simulink model "SVPWM_FOC"  (R2024a)
settings: Solver=ode23tb  StartTime=0.0  StopTime=1  MaxStep=0.00001  RelTol=1e-3
libraries: spsVoltageMeasurementLib x6, spsMosfetLib x6, slpidlib x3, spsDCVoltageSourceLib x2, spsPermanentMagnetSynchronousMachineLib x1, simulink x1, autolibpmsmexterior x1, spsUniversalBridgeLib x1, sps_lib x1
settings Model: Creator=hzn  LastModifiedBy=hzn

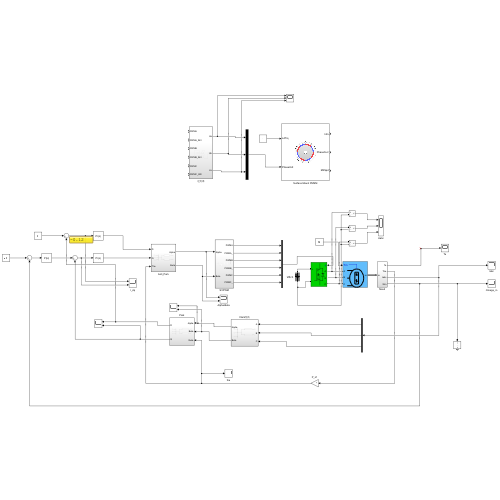
[thumbnail: Simulink's stored preview of the top-level diagram]
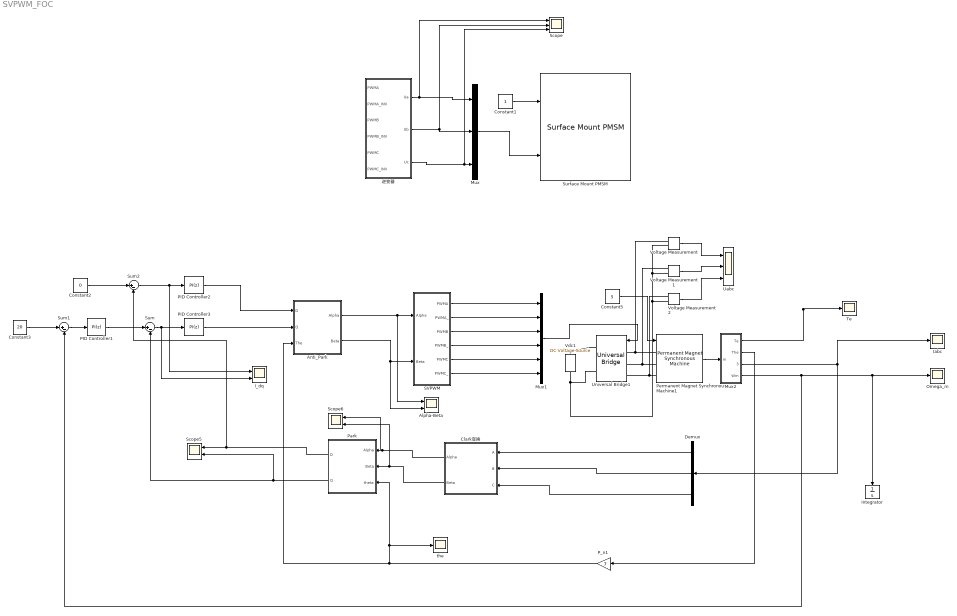
== system SVPWM_FOC ==
  Alpha-Beta : Scope  NumInputPorts=2
  Anti_Park : Subsystem
  Clark变换 : Subsystem
  Constant1 : Constant
  Constant2 : Constant  Value=0
  Constant3 : Constant  Value=20
  Constant5 : Constant  Value=5
  Demux : Demux  Outputs=3
  I_dq : Scope  NumInputPorts=2
  Iabc : Scope
  Integrator : Integrator
  Mux : Mux  Inputs=3
  Mux1 : Mux  Inputs=6
  Mux2 : Subsystem
  Omega_m : Scope
  PID Controller1 : slpidlib/PID Controller  Controller=PI  Form=Parallel  TimeDomain=Discrete-time  UseExternalTs=off  SampleTime=-1  IntegratorMethod=Forward Euler  FilterMethod=Forward Euler  ControllerParametersSource=internal  P=0.7  I=35  UseKiTs=off  D=0  UseExternalDerivativeSource=off  N=100  UseFilter=on  TunerSelectOption=Transfer Function Based (PID Tuner App)  InitialConditionSource=internal  InitialConditionForIntegrator=0  InitialConditionForFilter=0  DifferentiatorICPrevScaledInput=0  ExternalReset=none  TrackingMode=off  Kt=1  LimitOutput=off  SatLimitsSource=internal  UpperSaturationLimit=inf  LowerSaturationLimit=-inf  LinearizeAsGain=on  AntiWindupMode=none  Kb=1  LimitIntegrator=off  UpperIntegratorSaturationLimit=inf  LowerIntegratorSaturationLimit=-inf  POutMin=[]  POutMax=[]  IOutMin=[]  IOutMax=[]  DOutMin=[]  DOutMax=[]  NOutMin=[]  NOutMax=[]  SumOutMin=[]  SumOutMax=[]  SaturationOutMin=[]  SaturationOutMax=[]  PParamMin=[]  PParamMax=[]  IParamMin=[]  IParamMax=[]  DParamMin=[]  DParamMax=[]  NParamMin=[]  NParamMax=[]  KbParamMin=[]  KbParamMax=[]  KtParamMin=[]  KtParamMax=[]  KbOutMin=[]  KbOutMax=[]  KtOutMin=[]  KtOutMax=[]  IntegratorOutMin=[]  IntegratorOutMax=[]  FilterOutMin=[]  FilterOutMax=[]  SumI1OutMin=[]  SumI1OutMax=[]  SumI2OutMin=[]  SumI2OutMax=[]  SumI3OutMin=[]  SumI3OutMax=[]  SumI4OutMin=[]  SumI4OutMax=[]  SumDOutMin=[]  SumDOutMax=[]  DifferentiatorOutMin=[]  DifferentiatorOutMax=[]  FilterDiffOutCoefMin=[]  FilterDiffOutCoefMax=[]  ReciprocalOutMin=[]  ReciprocalOutMax=[]  SumDenOutMin=[]  SumDenOutMax=[]  SumNumOutMin=[]  SumNumOutMax=[]  DivideOutMin=[]  DivideOutMax=[]  UdiffTsProdOutMin=[]  UdiffTsProdOutMax=[]  NTsProdOutMin=[]  NTsProdOutMax=[]  UintegralTsProdOutMin=[]  UintegralTsProdOutMax=[]  UngainTsProdOutMin=[]  UngainTsProdOutMax=[]  ClampingZeroOutDataTypeStr=Inherit: Inherit via back propagation  ClampingZeroOutMin=[]  ClampingZeroOutMax=[]  FilterDenConstantOutDataTypeStr=Inherit: Inherit via back propagation  FilterDenConstantOutMin=[]  FilterDenConstantOutMax=[]  PCopyOutDataTypeStr=Inherit: Inherit via back propagation  PCopyOutMin=[]  PCopyOutMax=[]  NCopyOutDataTypeStr=Inherit: Inherit via back propagation  NCopyOutMin=[]  NCopyOutMax=[]  IntegratorContinuousStateAttributes=''  IntegratorStateMustResolveToSignalObject=off  IntegratorRTWStateStorageClass=Auto  FilterContinuousStateAttributes=''  FilterStateMustResolveToSignalObject=off  FilterRTWStateStorageClass=Auto  ParallelPVariant=InternalParameters  IdealPVariant=Disabled  IVariant=InternalParameters  DVariant=Disabled  IntegratorVariant=Discrete  SatVariant=Disabled  AWVariant=Passthrough  PCopyVariant=Disabled  TRVariant=Disabled  FdbkBlocksVariant=Forward  IdealPFdbkVariant=Disabled  SatFdbkVariant=Disabled  DerivativeFilterVariant=Disabled  NVariant=Disabled  NCopyVariant=Disabled_SignalSpec  FilterICVariant=Disabled  IntegratorICVariant=InternalICs  ExternalResetVariant=Disabled  TRSumVariant=Passthrough  SumFdbkVariant=Disabled  SumVariant=Sum_PI  TsampFilterVariant=InternalTs  TsampNgainVariant=Passthrough  TsampIntegralVariant=Disabled_SignalSpec  ExternalSaturationOutDataTypeStr=Inherit: Same as second input  DerivativeSourceVariant=Disabled
  PID Controller2 : slpidlib/PID Controller  Controller=PI  Form=Parallel  TimeDomain=Discrete-time  UseExternalTs=off  SampleTime=-1  IntegratorMethod=Forward Euler  FilterMethod=Forward Euler  ControllerParametersSource=internal  P=5  I=80  UseKiTs=off  D=0  UseExternalDerivativeSource=off  N=100  UseFilter=on  TunerSelectOption=Transfer Function Based (PID Tuner App)  InitialConditionSource=internal  InitialConditionForIntegrator=0  InitialConditionForFilter=0  DifferentiatorICPrevScaledInput=0  ExternalReset=none  TrackingMode=off  Kt=1  LimitOutput=off  SatLimitsSource=internal  UpperSaturationLimit=inf  LowerSaturationLimit=-inf  LinearizeAsGain=on  AntiWindupMode=none  Kb=1  LimitIntegrator=off  UpperIntegratorSaturationLimit=inf  LowerIntegratorSaturationLimit=-inf  POutMin=[]  POutMax=[]  IOutMin=[]  IOutMax=[]  DOutMin=[]  DOutMax=[]  NOutMin=[]  NOutMax=[]  SumOutMin=[]  SumOutMax=[]  SaturationOutMin=[]  SaturationOutMax=[]  PParamMin=[]  PParamMax=[]  IParamMin=[]  IParamMax=[]  DParamMin=[]  DParamMax=[]  NParamMin=[]  NParamMax=[]  KbParamMin=[]  KbParamMax=[]  KtParamMin=[]  KtParamMax=[]  KbOutMin=[]  KbOutMax=[]  KtOutMin=[]  KtOutMax=[]  IntegratorOutMin=[]  IntegratorOutMax=[]  FilterOutMin=[]  FilterOutMax=[]  SumI1OutMin=[]  SumI1OutMax=[]  SumI2OutMin=[]  SumI2OutMax=[]  SumI3OutMin=[]  SumI3OutMax=[]  SumI4OutMin=[]  SumI4OutMax=[]  SumDOutMin=[]  SumDOutMax=[]  DifferentiatorOutMin=[]  DifferentiatorOutMax=[]  FilterDiffOutCoefMin=[]  FilterDiffOutCoefMax=[]  ReciprocalOutMin=[]  ReciprocalOutMax=[]  SumDenOutMin=[]  SumDenOutMax=[]  SumNumOutMin=[]  SumNumOutMax=[]  DivideOutMin=[]  DivideOutMax=[]  UdiffTsProdOutMin=[]  UdiffTsProdOutMax=[]  NTsProdOutMin=[]  NTsProdOutMax=[]  UintegralTsProdOutMin=[]  UintegralTsProdOutMax=[]  UngainTsProdOutMin=[]  UngainTsProdOutMax=[]  ClampingZeroOutDataTypeStr=Inherit: Inherit via back propagation  ClampingZeroOutMin=[]  ClampingZeroOutMax=[]  FilterDenConstantOutDataTypeStr=Inherit: Inherit via back propagation  FilterDenConstantOutMin=[]  FilterDenConstantOutMax=[]  PCopyOutDataTypeStr=Inherit: Inherit via back propagation  PCopyOutMin=[]  PCopyOutMax=[]  NCopyOutDataTypeStr=Inherit: Inherit via back propagation  NCopyOutMin=[]  NCopyOutMax=[]  IntegratorContinuousStateAttributes=''  IntegratorStateMustResolveToSignalObject=off  IntegratorRTWStateStorageClass=Auto  FilterContinuousStateAttributes=''  FilterStateMustResolveToSignalObject=off  FilterRTWStateStorageClass=Auto  ParallelPVariant=InternalParameters  IdealPVariant=Disabled  IVariant=InternalParameters  DVariant=Disabled  IntegratorVariant=Discrete  SatVariant=Disabled  AWVariant=Passthrough  PCopyVariant=Disabled  TRVariant=Disabled  FdbkBlocksVariant=Forward  IdealPFdbkVariant=Disabled  SatFdbkVariant=Disabled  DerivativeFilterVariant=Disabled  NVariant=Disabled  NCopyVariant=Disabled_SignalSpec  FilterICVariant=Disabled  IntegratorICVariant=InternalICs  ExternalResetVariant=Disabled  TRSumVariant=Passthrough  SumFdbkVariant=Disabled  SumVariant=Sum_PI  TsampFilterVariant=InternalTs  TsampNgainVariant=Passthrough  TsampIntegralVariant=Disabled_SignalSpec  ExternalSaturationOutDataTypeStr=Inherit: Same as second input  DerivativeSourceVariant=Disabled
  PID Controller3 : slpidlib/PID Controller  Controller=PI  Form=Parallel  TimeDomain=Discrete-time  UseExternalTs=off  SampleTime=-1  IntegratorMethod=Forward Euler  FilterMethod=Forward Euler  ControllerParametersSource=internal  P=5  I=80  UseKiTs=off  D=0  UseExternalDerivativeSource=off  N=100  UseFilter=on  TunerSelectOption=Transfer Function Based (PID Tuner App)  InitialConditionSource=internal  InitialConditionForIntegrator=0  InitialConditionForFilter=0  DifferentiatorICPrevScaledInput=0  ExternalReset=none  TrackingMode=off  Kt=1  LimitOutput=off  SatLimitsSource=internal  UpperSaturationLimit=inf  LowerSaturationLimit=-inf  LinearizeAsGain=on  AntiWindupMode=none  Kb=1  LimitIntegrator=off  UpperIntegratorSaturationLimit=inf  LowerIntegratorSaturationLimit=-inf  POutMin=[]  POutMax=[]  IOutMin=[]  IOutMax=[]  DOutMin=[]  DOutMax=[]  NOutMin=[]  NOutMax=[]  SumOutMin=[]  SumOutMax=[]  SaturationOutMin=[]  SaturationOutMax=[]  PParamMin=[]  PParamMax=[]  IParamMin=[]  IParamMax=[]  DParamMin=[]  DParamMax=[]  NParamMin=[]  NParamMax=[]  KbParamMin=[]  KbParamMax=[]  KtParamMin=[]  KtParamMax=[]  KbOutMin=[]  KbOutMax=[]  KtOutMin=[]  KtOutMax=[]  IntegratorOutMin=[]  IntegratorOutMax=[]  FilterOutMin=[]  FilterOutMax=[]  SumI1OutMin=[]  SumI1OutMax=[]  SumI2OutMin=[]  SumI2OutMax=[]  SumI3OutMin=[]  SumI3OutMax=[]  SumI4OutMin=[]  SumI4OutMax=[]  SumDOutMin=[]  SumDOutMax=[]  DifferentiatorOutMin=[]  DifferentiatorOutMax=[]  FilterDiffOutCoefMin=[]  FilterDiffOutCoefMax=[]  ReciprocalOutMin=[]  ReciprocalOutMax=[]  SumDenOutMin=[]  SumDenOutMax=[]  SumNumOutMin=[]  SumNumOutMax=[]  DivideOutMin=[]  DivideOutMax=[]  UdiffTsProdOutMin=[]  UdiffTsProdOutMax=[]  NTsProdOutMin=[]  NTsProdOutMax=[]  UintegralTsProdOutMin=[]  UintegralTsProdOutMax=[]  UngainTsProdOutMin=[]  UngainTsProdOutMax=[]  ClampingZeroOutDataTypeStr=Inherit: Inherit via back propagation  ClampingZeroOutMin=[]  ClampingZeroOutMax=[]  FilterDenConstantOutDataTypeStr=Inherit: Inherit via back propagation  FilterDenConstantOutMin=[]  FilterDenConstantOutMax=[]  PCopyOutDataTypeStr=Inherit: Inherit via back propagation  PCopyOutMin=[]  PCopyOutMax=[]  NCopyOutDataTypeStr=Inherit: Inherit via back propagation  NCopyOutMin=[]  NCopyOutMax=[]  IntegratorContinuousStateAttributes=''  IntegratorStateMustResolveToSignalObject=off  IntegratorRTWStateStorageClass=Auto  FilterContinuousStateAttributes=''  FilterStateMustResolveToSignalObject=off  FilterRTWStateStorageClass=Auto  ParallelPVariant=InternalParameters  IdealPVariant=Disabled  IVariant=InternalParameters  DVariant=Disabled  IntegratorVariant=Discrete  SatVariant=Disabled  AWVariant=Passthrough  PCopyVariant=Disabled  TRVariant=Disabled  FdbkBlocksVariant=Forward  IdealPFdbkVariant=Disabled  SatFdbkVariant=Disabled  DerivativeFilterVariant=Disabled  NVariant=Disabled  NCopyVariant=Disabled_SignalSpec  FilterICVariant=Disabled  IntegratorICVariant=InternalICs  ExternalResetVariant=Disabled  TRSumVariant=Passthrough  SumFdbkVariant=Disabled  SumVariant=Sum_PI  TsampFilterVariant=InternalTs  TsampNgainVariant=Passthrough  TsampIntegralVariant=Disabled_SignalSpec  ExternalSaturationOutDataTypeStr=Inherit: Same as second input  DerivativeSourceVariant=Disabled
  P_n1 : Gain  Gain=7
  Park : Subsystem
  Permanent Magnet Synchronous Machine1 : spsPermanentMagnetSynchronousMachineLib/Permanent Magnet Synchronous Machine  NbPhases=3  FluxDistribution=Sinusoidal  RotorType=Round  MechanicalLoad=Torque Tm  PresetModel=No  ShowDetailedParameters=on  MeasurementBus=off  Resistance=0.958  Inductance=8.5e-3  dqInductances=[5.25e-3,12e-3]  La=0.000835  MachineConstant=Flux linkage established by magnets (V.s)  Flux=0.1827  VoltageCst=231.9668  TorqueCst=1.9184  Flat=120  Mechanical=[0.003 0.008 7]  PolePairs=3  InitialConditions=[0,0, 0,0]  InitialConditions5ph=[0 0 0 0 0 0]  RefAngle=Aligned with phase A axis (original Park)  IterativeDiscreteModel=Trapezoidal non iterative  TsBlock=-1  TsPowergui=0
  SVPWM : Subsystem
  Scope : Scope  NumInputPorts=3
  Scope5 : Scope  NumInputPorts=2
  Scope6 : Scope  NumInputPorts=2
  Sum : Sum  Inputs=|+-
  Sum1 : Sum  Inputs=|+-
  Sum2 : Sum  Inputs=|+-
  Surface Mount PMSM : autolibpmsmexterior/Surface Mount PMSM  port_config=Torque  sim_type=Continuous  Ts=0.001  FilePath=E:\Sandbox\Bauto\Work\surfacepmsm_motordata.m  P=7  Rs=0.12  Ldq_=3.752e-4  KConstText=Permanent flux linkage constant (lambda_pm):  lambda_pm=0.1194  Ke=159.9771  Kt=1.323  mechanical=[0.0027, 4.924e-4, 0]  idq0=[0 0]  theta_init=0  omega_init=0  KConst=0.1194  lambda_pm_calc=0.1194  RefBlkName='autolibpmsmexterior/Surface Mount PMSM'  aMode=1  Ldq="[0.0003752   0.0003752]"
      settings: LibrarySourceBlock=autolibemachines/Surface Mount PMSM
  Te : Scope
  Uabc : Scope  NumInputPorts=3
  Universal Bridge1 : spsUniversalBridgeLib/Universal Bridge  Arms=3  SnubberResistance=1e5  SnubberCapacitance=inf  Device=MOSFET / Diodes  Ron=1e-3  Lon=0  ForwardVoltages="[  0  0  ]"  ForwardVoltage=0  GTOparameters=[ 10e-6 , 20e-6 ]  IGBTparameters=[ 1e-6 , 2e-6 ]  Measurements=None  Measurements_2=None  converterType=Rectifier
  Vdc1 : spsDCVoltageSourceLib/DC Voltage Source  Amplitude=100  Measurements=None
  Voltage Measurement : spsVoltageMeasurementLib/Voltage Measurement  PhasorSimulation=off  OutputType=Complex  PSBequivalent=0
  Voltage Measurement1 : spsVoltageMeasurementLib/Voltage Measurement  PhasorSimulation=off  OutputType=Complex  PSBequivalent=0
  Voltage Measurement2 : spsVoltageMeasurementLib/Voltage Measurement  PhasorSimulation=off  OutputType=Complex  PSBequivalent=0
  the : Scope
  逆变器 : Subsystem
  wires:
  Clark变换/1(Alpha) -> Scope6/1, Park/1(Alpha)
  Clark变换/2(Beta) -> Scope6/2, Park/2(Beta)
  SVPWM/1(PWMA) -> Mux1/1
  SVPWM/2(PWMA_) -> Mux1/2
  SVPWM/3(PWMB) -> Mux1/3
  SVPWM/4(PWMB_) -> Mux1/4
  SVPWM/5(PWMC) -> Mux1/5
  SVPWM/6(PWMC_) -> Mux1/6
  Mux2/3(Iabc) -> Iabc/1, Demux/1
  Demux/1 -> Clark变换/1(A)
  Demux/2 -> Clark变换/2(B)
  Demux/3 -> Clark变换/3(C)
  P_n1/1 -> the/1, Park/3(theta), Anti_Park/3(The)
  Park/2(Q) -> Sum/2, Scope5/2
  PID Controller1/1 -> Sum/1
  Sum1/1 -> PID Controller1/1
  Constant3/1 -> Sum1/1
  Constant2/1 -> Sum2/1
  Sum2/1 -> I_dq/1, PID Controller2/1
  PID Controller2/1 -> Anti_Park/1(D)
  Park/1(D) -> Sum2/2, Scope5/1
  PID Controller3/1 -> Anti_Park/2(Q)
  Mux/1 -> Surface Mount PMSM/2
  Constant1/1 -> Surface Mount PMSM/1
  逆变器/3(Uc) -> Scope/3, Mux/3
  逆变器/1(Ua) -> Scope/1, Mux/1
  逆变器/2(Ub) -> Mux/2, Scope/2
  Mux1/1 -> Universal Bridge1/1
  Permanent Magnet Synchronous Machine1/1 -> Mux2/1(m)
  Constant5/1 -> Permanent Magnet Synchronous Machine1/1
  Sum/1 -> I_dq/2, PID Controller3/1
  Mux2/2(The) -> P_n1/1
  Anti_Park/2(Beta) -> SVPWM/2(Beta), Alpha-Beta/2
  Anti_Park/1(Alpha) -> Alpha-Beta/1, SVPWM/1(Alpha)
  Voltage Measurement/1 -> Uabc/1
  Voltage Measurement1/1 -> Uabc/2
  Voltage Measurement2/1 -> Uabc/3
  Mux2/1(Te) -> Te/1
  Mux2/4(Wm) -> Sum1/2, Integrator/1, Omega_m/1
  connections:
  Universal Bridge1/RConn1 -- Vdc1/RConn1
  Universal Bridge1/RConn2 -- Voltage Measurement1/LConn2 -- Voltage Measurement/LConn2 -- Voltage Measurement2/LConn2 -- Vdc1/LConn1
  Permanent Magnet Synchronous Machine1/LConn1 -- Voltage Measurement/LConn1 -- Universal Bridge1/LConn1
  Permanent Magnet Synchronous Machine1/LConn2 -- Voltage Measurement1/LConn1 -- Universal Bridge1/LConn2
  Permanent Magnet Synchronous Machine1/LConn3 -- Voltage Measurement2/LConn1 -- Universal Bridge1/LConn3

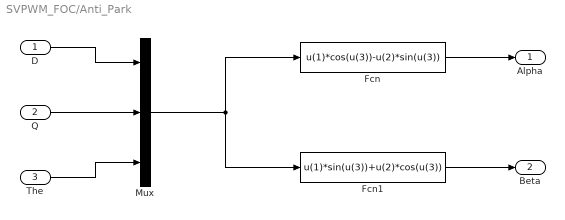
== system SVPWM_FOC/Anti_Park ==
  D : Inport
  Q : Inport  Port=2
  The : Inport  Port=3
  Fcn : Fcn  Expr=u(1)*cos(u(3))-u(2)*sin(u(3))
  Fcn1 : Fcn  Expr=u(1)*sin(u(3))+u(2)*cos(u(3))
  Mux : Mux  Inputs=3
  Alpha : Outport
  Beta : Outport  Port=2
  wires:
  D/1 -> Mux/1
  Q/1 -> Mux/2
  The/1 -> Mux/3
  Mux/1 -> Fcn1/1, Fcn/1
  Fcn1/1 -> Beta/1
  Fcn/1 -> Alpha/1

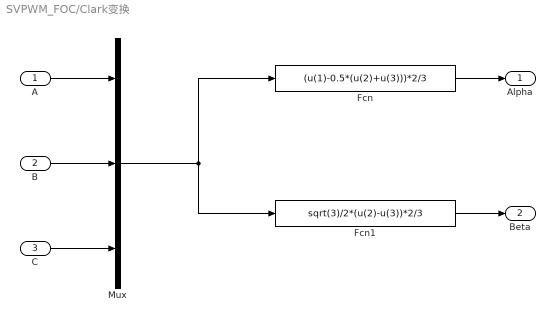
== system SVPWM_FOC/Clark变换 ==
  A : Inport
  B : Inport  Port=2
  C : Inport  Port=3
  Fcn : Fcn  Expr=(u(1)-0.5*(u(2)+u(3)))*2/3
  Fcn1 : Fcn  Expr=sqrt(3)/2*(u(2)-u(3))*2/3
  Mux : Mux  Inputs=3
  Alpha : Outport
  Beta : Outport  Port=2
  wires:
  B/1 -> Mux/2
  A/1 -> Mux/1
  C/1 -> Mux/3
  Mux/1 -> Fcn1/1, Fcn/1
  Fcn/1 -> Alpha/1
  Fcn1/1 -> Beta/1

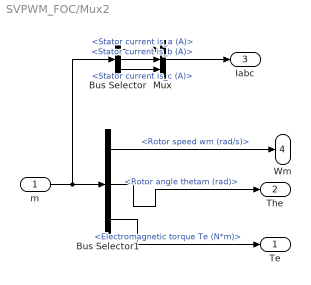
== system SVPWM_FOC/Mux2 ==
  m : Inport
  Bus Selector : BusSelector  OutputSignals=Stator current is_a (A),Stator current is_b (A),Stator current is_c (A)
  Bus Selector1 : BusSelector  OutputSignals=Rotor speed wm (rad/s),Rotor angle thetam (rad),Electromagnetic torque Te (N*m)
  Mux : Mux  Inputs=3
  Te : Outport
  The : Outport  Port=2
  Iabc : Outport  Port=3
  Wm : Outport  Port=4
  wires:
  Bus Selector1/1 -> Wm/1  "<Rotor speed wm (rad/s)>"
  Bus Selector1/2 -> The/1  "<Rotor angle thetam (rad)>"
  Bus Selector1/3 -> Te/1  "<Electromagnetic torque Te (N*m)>"
  m/1 -> Bus Selector/1, Bus Selector1/1
  Bus Selector/2 -> Mux/2  "<Stator current is_b (A)>"
  Bus Selector/3 -> Mux/3  "<Stator current is_c (A)>"
  Bus Selector/1 -> Mux/1  "<Stator current is_a (A)>"
  Mux/1 -> Iabc/1

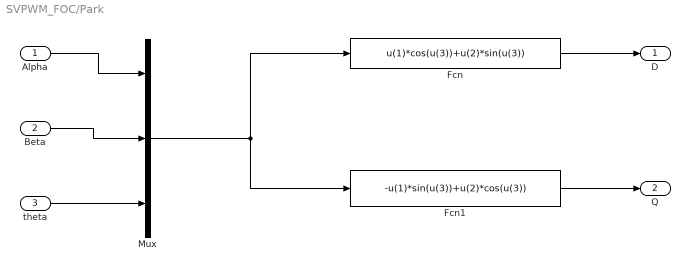
== system SVPWM_FOC/Park ==
  Alpha : Inport
  Beta : Inport  Port=2
  theta : Inport  Port=3
  Fcn : Fcn  Expr=u(1)*cos(u(3))+u(2)*sin(u(3))
  Fcn1 : Fcn  Expr=-u(1)*sin(u(3))+u(2)*cos(u(3))
  Mux : Mux  Inputs=3
  D : Outport
  Q : Outport  Port=2
  wires:
  Alpha/1 -> Mux/1
  Beta/1 -> Mux/2
  theta/1 -> Mux/3
  Mux/1 -> Fcn/1, Fcn1/1
  Fcn/1 -> D/1
  Fcn1/1 -> Q/1

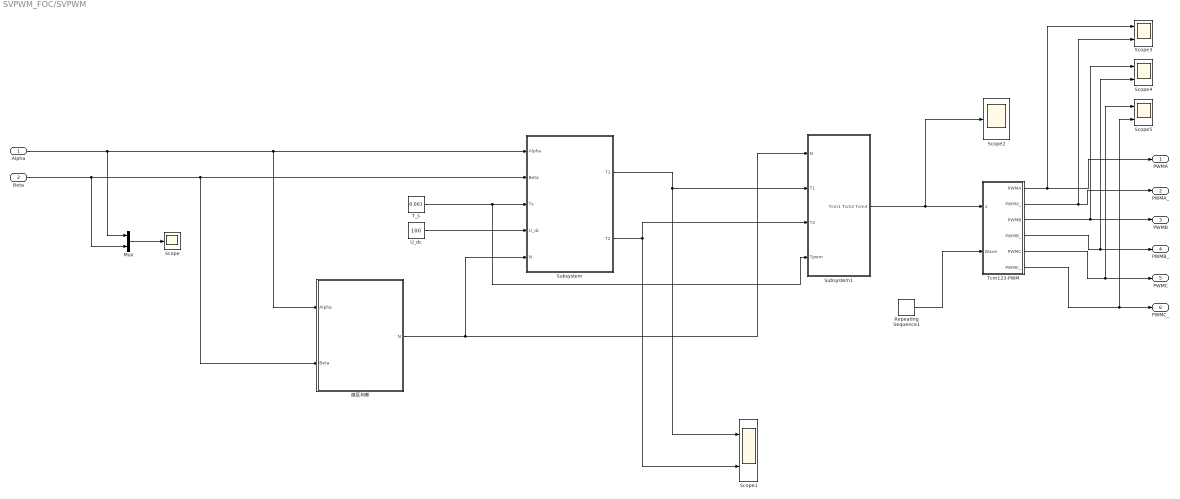
== system SVPWM_FOC/SVPWM ==
  Alpha : Inport
  Beta : Inport  Port=2
  Mux : Mux  Inputs=2
  Repeating Sequence1 : simulink/Sources/Repeating Sequence  rep_seq_t=[0 0.001/2 0.001]  rep_seq_y=[0 0.001/2 0]
  Scope : Scope
  Scope{1,3..5} (4 alike) : Scope  NumInputPorts=2
  Scope2 : Scope
  Subsystem : Subsystem
  Subsystem1 : Subsystem
  T_s : Constant  Value=0.001
  Tcm123-PWM : Subsystem
  U_dc : Constant  Value=100
  扇区判断 : Subsystem
  PWMA : Outport
  PWMA_ : Outport  Port=2
  PWMB : Outport  Port=3
  PWMB_ : Outport  Port=4
  PWMC : Outport  Port=5
  PWMC_ : Outport  Port=6
  wires:
  U_dc/1 -> Subsystem/4(U_dc)
  Subsystem/1(T1) -> Scope1/1, Subsystem1/2(T1)
  Subsystem/2(T2) -> Scope1/2, Subsystem1/3(T2)
  Alpha/1 -> Mux/1, Subsystem/1(Alpha), 扇区判断/1(Alpha)
  Mux/1 -> Scope/1
  Beta/1 -> Mux/2, Subsystem/2(Beta), 扇区判断/2(Beta)
  扇区判断/1(N) -> Subsystem/5(N), Subsystem1/1(N)
  T_s/1 -> Subsystem1/4(Tpwm), Subsystem/3(Ts)
  Subsystem1/1(Tcm1 Tcm2 Tcm3) -> Scope2/1, Tcm123-PWM/1(Tcm123)
  Repeating Sequence1/1 -> Tcm123-PWM/2(Wave)
  Tcm123-PWM/3(PWMB) -> Scope4/1, PWMB/1
  Tcm123-PWM/4(PWMB_) -> Scope4/2, PWMB_/1
  Tcm123-PWM/5(PWMC) -> Scope5/1, PWMC/1
  Tcm123-PWM/6(PWMC_) -> Scope5/2, PWMC_/1
  Tcm123-PWM/1(PWMA) -> Scope3/1, PWMA/1
  Tcm123-PWM/2(PWMA_) -> Scope3/2, PWMA_/1

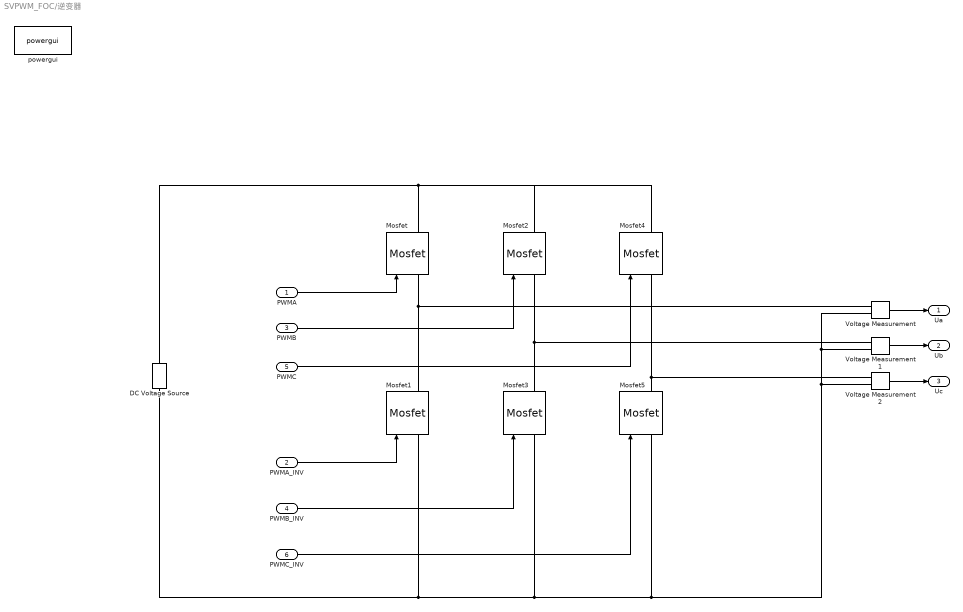
== system SVPWM_FOC/逆变器 ==
  PWMA : Inport
  PWMA_INV : Inport  Port=2
  PWMB : Inport  Port=3
  PWMB_INV : Inport  Port=4
  PWMC : Inport  Port=5
  PWMC_INV : Inport  Port=6
  DC Voltage Source : spsDCVoltageSourceLib/DC Voltage Source  Amplitude=100  Measurements=None
  Mosfet{,1..5} (6 alike) : spsMosfetLib/Mosfet  Ron=0.1  Lon=0  Rd=0.01  Vfd=0  IC=0  Rs=1e5  Cs=inf  Measurements=on
  Voltage Measurement : spsVoltageMeasurementLib/Voltage Measurement  PhasorSimulation=off  OutputType=Complex  PSBequivalent=0
  Voltage Measurement1 : spsVoltageMeasurementLib/Voltage Measurement  PhasorSimulation=off  OutputType=Complex  PSBequivalent=0
  Voltage Measurement2 : spsVoltageMeasurementLib/Voltage Measurement  PhasorSimulation=off  OutputType=Complex  PSBequivalent=0
  powergui : sps_lib/powergui  Priority=1  SimulationMode=Continuous  SampleTime=50e-6  frequency=60  Iterations=50  frequencyindice=0  Pbase=100e6  ErrMax=1e-4  UnitsV=kV  UnitsW=MW  buscounter=0  FunctionMessages=off  echomessages=off  EnableUseOfTLC=off  CurrentSourceSwitches=off  DisableSnubberDevices=off  DisableRonSwitches=off  DisableVfSwitches=off  DisplayEquations=off  AutomaticDiscreteSolvers=off  SolverType=Tustin/Backward Euler (TBE)  Interpol=off  ExternalGateDelay=off  methode=off  Ts=100  x0status=blocks  SPID=on  SwTol=0  HookPort=off  NonlinearTolerance=1e-4  nMaxIteration=100  ContinueOnMaxIteration=off  RestoreLinks=warning  ResistiveCurrentMeasurement=off  Frange=[0:2:500]  Ylog=off  Xlog=on  ShowGrid=off  save=off  variable=ZData  structure=0  ZoomFFT=off  StartTime=0.0  cycles=1  DisplayStyle=1  fundamental=60  FreqAxis=off  MaxFrequency=1000  frequencyindicesteady=1  RmsSteady=1  display=off
  Ua : Outport
  Ub : Outport  Port=2
  Uc : Outport  Port=3
  wires:
  PWMA/1 -> Mosfet/1
  PWMA_INV/1 -> Mosfet1/1
  PWMB/1 -> Mosfet2/1
  PWMC/1 -> Mosfet4/1
  PWMB_INV/1 -> Mosfet3/1
  PWMC_INV/1 -> Mosfet5/1
  Voltage Measurement/1 -> Ua/1
  Voltage Measurement1/1 -> Ub/1
  Voltage Measurement2/1 -> Uc/1
  connections:
  Mosfet/LConn1 -- Voltage Measurement/LConn1 -- Mosfet1/RConn1
  Mosfet2/LConn1 -- Voltage Measurement1/LConn1 -- Mosfet3/RConn1
  Mosfet4/LConn1 -- Voltage Measurement2/LConn1 -- Mosfet5/RConn1
  Voltage Measurement/LConn2 -- Voltage Measurement1/LConn2 -- Mosfet3/LConn1 -- DC Voltage Source/LConn1 -- Mosfet1/LConn1 -- Mosfet5/LConn1 -- Voltage Measurement2/LConn2
  DC Voltage Source/RConn1 -- Mosfet/RConn1 -- Mosfet2/RConn1 -- Mosfet4/RConn1

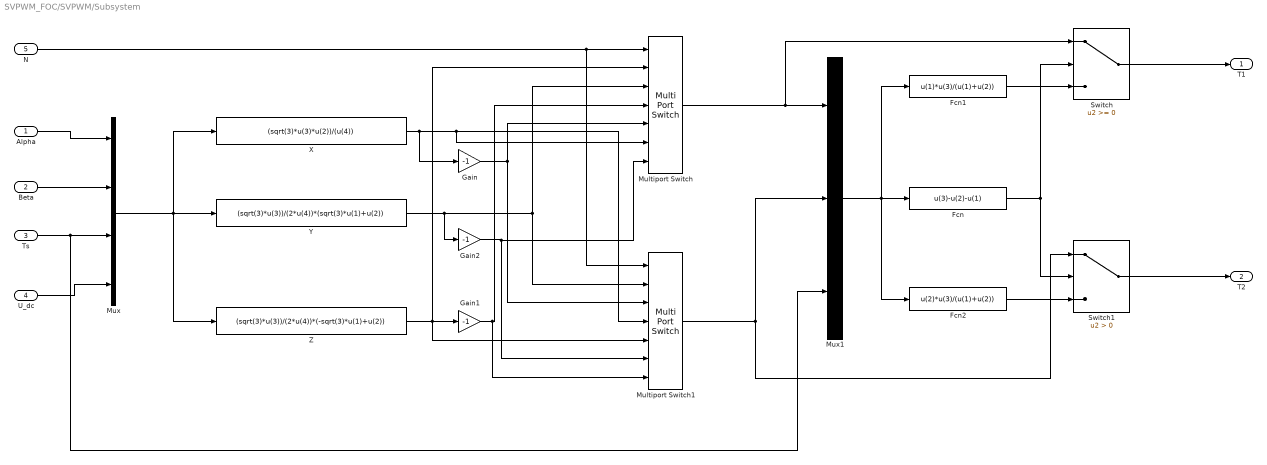
== system SVPWM_FOC/SVPWM/Subsystem ==
  Alpha : Inport
  Beta : Inport  Port=2
  Ts : Inport  Port=3
  U_dc : Inport  Port=4
  N : Inport  Port=5
  Fcn : Fcn  Expr=u(3)-u(2)-u(1)
  Fcn1 : Fcn  Expr=u(1)*u(3)/(u(1)+u(2))
  Fcn2 : Fcn  Expr=u(2)*u(3)/(u(1)+u(2))
  Gain : Gain  Gain=-1
  Gain1 : Gain  Gain=-1
  Gain2 : Gain  Gain=-1
  Multiport Switch : MultiPortSwitch  Inputs=6  SaturateOnIntegerOverflow=off  InputSameDT=off
  Multiport Switch1 : MultiPortSwitch  Inputs=6  SaturateOnIntegerOverflow=off  InputSameDT=off
  Mux : Mux
  Mux1 : Mux  Inputs=3
  Switch : Switch  SaturateOnIntegerOverflow=off  InputSameDT=off
  Switch1 : Switch  Criteria=u2 > Threshold  SaturateOnIntegerOverflow=off  InputSameDT=off
  X : Fcn  Expr=(sqrt(3)*u(3)*u(2))/(u(4))
  Y : Fcn  Expr=(sqrt(3)*u(3))/(2*u(4))*(sqrt(3)*u(1)+u(2))
  Z : Fcn  Expr=(sqrt(3)*u(3))/(2*u(4))*(-sqrt(3)*u(1)+u(2))
  T1 : Outport
  T2 : Outport  Port=2
  wires:
  Alpha/1 -> Mux/1
  Beta/1 -> Mux/2
  U_dc/1 -> Mux/4
  Mux/1 -> X/1, Z/1, Y/1
  Y/1 -> Gain2/1, Multiport Switch1/2, Multiport Switch/3
  Z/1 -> Multiport Switch1/5, Gain1/1, Multiport Switch/2
  X/1 -> Multiport Switch/6, Multiport Switch1/4, Gain/1
  N/1 -> Multiport Switch1/1, Multiport Switch/1
  Gain/1 -> Multiport Switch1/3, Multiport Switch/5
  Gain1/1 -> Multiport Switch1/7, Multiport Switch/4
  Gain2/1 -> Multiport Switch1/6, Multiport Switch/7
  Multiport Switch/1 -> Switch/1, Mux1/1
  Ts/1 -> Mux1/3, Mux/3
  Mux1/1 -> Fcn2/1, Fcn1/1, Fcn/1
  Fcn1/1 -> Switch/3
  Fcn/1 -> Switch/2, Switch1/2
  Multiport Switch1/1 -> Mux1/2, Switch1/1
  Fcn2/1 -> Switch1/3
  Switch/1 -> T1/1
  Switch1/1 -> T2/1

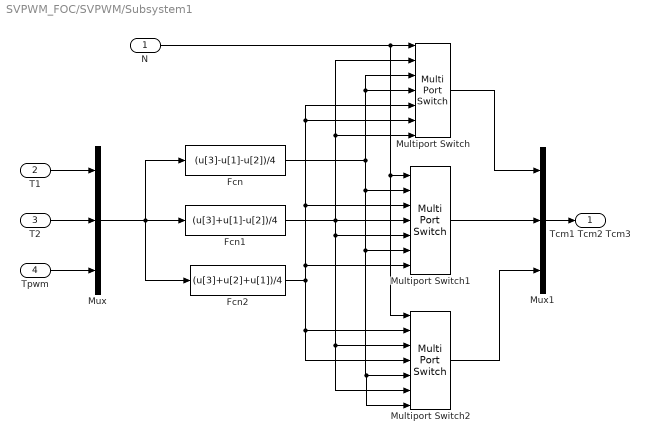
== system SVPWM_FOC/SVPWM/Subsystem1 ==
  N : Inport
  T1 : Inport  Port=2
  T2 : Inport  Port=3
  Tpwm : Inport  Port=4
  Fcn : Fcn  Expr=(u[3]-u[1]-u[2])/4
  Fcn1 : Fcn  Expr=(u[3]+u[1]-u[2])/4
  Fcn2 : Fcn  Expr=(u[3]+u[2]+u[1])/4
  Multiport Switch : MultiPortSwitch  Inputs=6  SaturateOnIntegerOverflow=off  InputSameDT=off
  Multiport Switch1 : MultiPortSwitch  Inputs=6  SaturateOnIntegerOverflow=off  InputSameDT=off
  Multiport Switch2 : MultiPortSwitch  Inputs=6  SaturateOnIntegerOverflow=off  InputSameDT=off
  Mux : Mux  Inputs=3
  Mux1 : Mux  Inputs=3
  Tcm1 Tcm2 Tcm3 : Outport
  wires:
  Fcn/1 -> Multiport Switch/3, Multiport Switch/4, Multiport Switch1/6, Multiport Switch2/5, Multiport Switch2/7, Multiport Switch1/2
  Mux/1 -> Fcn2/1, Fcn/1, Fcn1/1
  Multiport Switch/1 -> Mux1/1
  Multiport Switch2/1 -> Mux1/3
  Multiport Switch1/1 -> Mux1/2
  Mux1/1 -> Tcm1 Tcm2 Tcm3/1
  T2/1 -> Mux/2
  N/1 -> Multiport Switch2/1, Multiport Switch1/1, Multiport Switch/1
  Fcn2/1 -> Multiport Switch/5, Multiport Switch/6, Multiport Switch1/3, Multiport Switch1/7, Multiport Switch2/2, Multiport Switch2/4
  Tpwm/1 -> Mux/3
  Fcn1/1 -> Multiport Switch1/5, Multiport Switch2/3, Multiport Switch2/6, Multiport Switch1/4, Multiport Switch/7, Multiport Switch/2
  T1/1 -> Mux/1

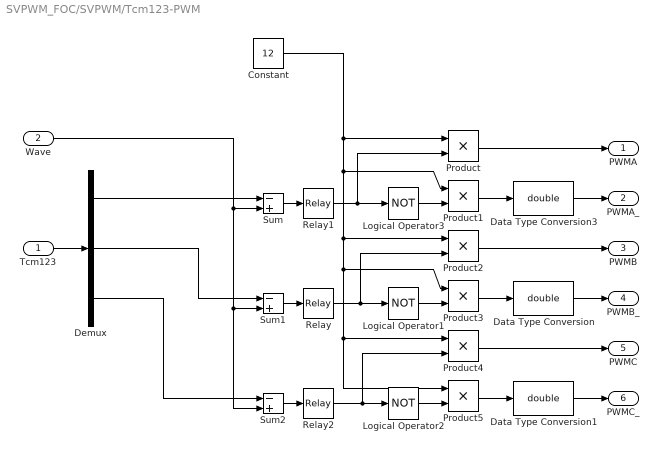
== system SVPWM_FOC/SVPWM/Tcm123-PWM ==
  Tcm123 : Inport
  Wave : Inport  Port=2
  Constant : Constant  Value=12
  Data Type Conversion : DataTypeConversion  OutDataTypeStr=double  SaturateOnIntegerOverflow=off  RndMeth=Floor
  Data Type Conversion1 : DataTypeConversion  OutDataTypeStr=double  SaturateOnIntegerOverflow=off  RndMeth=Floor
  Data Type Conversion3 : DataTypeConversion  OutDataTypeStr=double  SaturateOnIntegerOverflow=off  RndMeth=Floor
  Demux : Demux  Outputs=3
  Logical Operator1 : Logic  Operator=NOT  AllPortsSameDT=off  OutDataTypeStr=boolean
  Logical Operator2 : Logic  Operator=NOT  AllPortsSameDT=off  OutDataTypeStr=boolean
  Logical Operator3 : Logic  Operator=NOT  AllPortsSameDT=off  OutDataTypeStr=boolean
  Product{,1..5} (6 alike) : Product
  Relay : Relay  OffSwitchValue=-eps
  Relay1 : Relay  OffSwitchValue=-eps
  Relay2 : Relay  OffSwitchValue=-eps
  Sum : Sum  Inputs=-+  SaturateOnIntegerOverflow=on
  Sum1 : Sum  Inputs=-+  SaturateOnIntegerOverflow=on
  Sum2 : Sum  Inputs=-+  SaturateOnIntegerOverflow=on
  PWMA : Outport
  PWMA_ : Outport  Port=2
  PWMB : Outport  Port=3
  PWMB_ : Outport  Port=4
  PWMC : Outport  Port=5
  PWMC_ : Outport  Port=6
  wires:
  Tcm123/1 -> Demux/1
  Demux/3 -> Sum2/1
  Demux/2 -> Sum1/1
  Demux/1 -> Sum/1
  Wave/1 -> Sum1/2, Sum2/2, Sum/2
  Sum/1 -> Relay1/1
  Sum2/1 -> Relay2/1
  Sum1/1 -> Relay/1
  Relay1/1 -> Product/2, Logical Operator3/1
  Relay2/1 -> Product4/2, Logical Operator2/1
  Relay/1 -> Product2/2, Logical Operator1/1
  Logical Operator3/1 -> Product1/2
  Logical Operator1/1 -> Product3/2
  Logical Operator2/1 -> Product5/2
  Data Type Conversion3/1 -> PWMA_/1
  Data Type Conversion/1 -> PWMB_/1
  Data Type Conversion1/1 -> PWMC_/1
  Product1/1 -> Data Type Conversion3/1
  Product3/1 -> Data Type Conversion/1
  Product5/1 -> Data Type Conversion1/1
  Product/1 -> PWMA/1
  Product2/1 -> PWMB/1
  Product4/1 -> PWMC/1
  Constant/1 -> Product/1, Product1/1, Product2/1, Product4/1, Product5/1, Product3/1

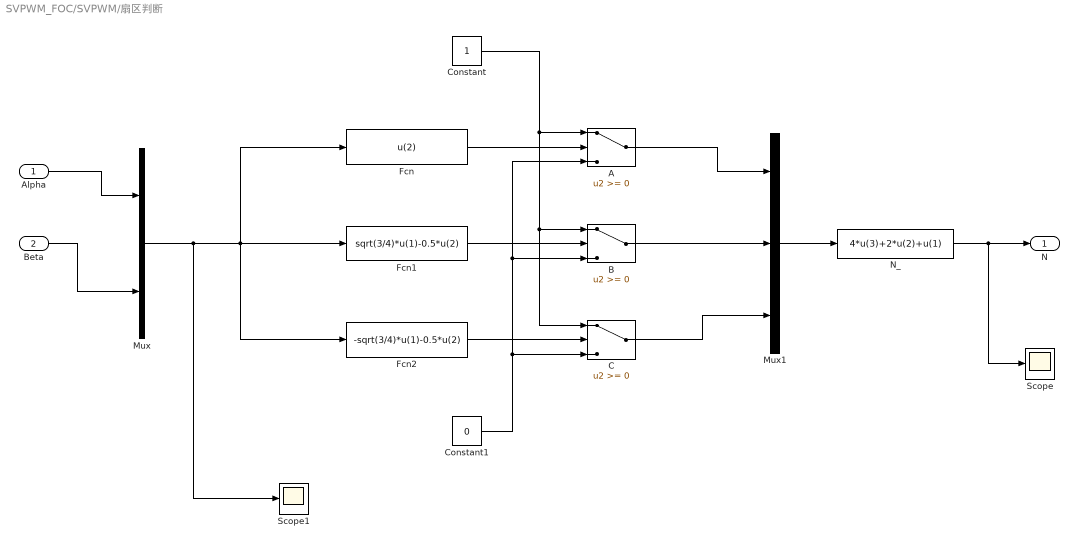
== system SVPWM_FOC/SVPWM/扇区判断 ==
  Alpha : Inport
  Beta : Inport  Port=2
  A : Switch  SaturateOnIntegerOverflow=off  InputSameDT=off
  B : Switch  SaturateOnIntegerOverflow=off  InputSameDT=off
  C : Switch  SaturateOnIntegerOverflow=off  InputSameDT=off
  Constant : Constant
  Constant1 : Constant  Value=0
  Fcn : Fcn  Expr=u(2)
  Fcn1 : Fcn  Expr=sqrt(3/4)*u(1)-0.5*u(2)
  Fcn2 : Fcn  Expr=-sqrt(3/4)*u(1)-0.5*u(2)
  Mux : Mux  Inputs=2
  Mux1 : Mux  Inputs=3
  N_ : Fcn  Expr=4*u(3)+2*u(2)+u(1)
  Scope : Scope
  Scope1 : Scope
  N : Outport
  wires:
  Alpha/1 -> Mux/1
  Beta/1 -> Mux/2
  Mux/1 -> Scope1/1, Fcn2/1, Fcn1/1, Fcn/1
  Fcn/1 -> A/2
  Fcn1/1 -> B/2
  Fcn2/1 -> C/2
  Constant/1 -> C/1, B/1, A/1
  Constant1/1 -> C/3, A/3, B/3
  A/1 -> Mux1/1
  B/1 -> Mux1/2
  C/1 -> Mux1/3
  Mux1/1 -> N_/1
  N_/1 -> Scope/1, N/1
